simulink model "avoidance"  (R2022a)
settings: Solver=FixedStepAuto  StartTime=0.0  StopTime=15  FixedStep=0.01  RelTol=1e-3
values from neighbouring files (symbols this model uses):
  a10 = pi/4    (= 0.785398163397)    [gen_data.m]
  a20 = 3*pi/4    (= 2.35619449019)    [gen_data.m]
  x10 = x0(i,1)    [gen_data.m]
  x20 = 10+x0(i,2)    [gen_data.m]
  y10 = x0(i,3)    [gen_data.m]
  y20 = x0(i,4)    [gen_data.m]
  z0 = 0    [gen_data.m]
settings Model: Creator=diego  LastModifiedBy=diego

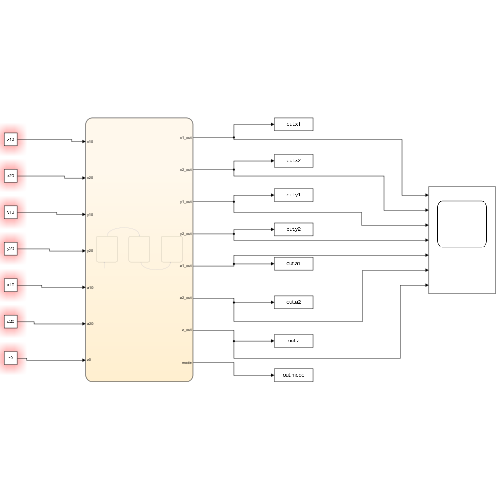
[thumbnail: Simulink's stored preview of the top-level diagram]
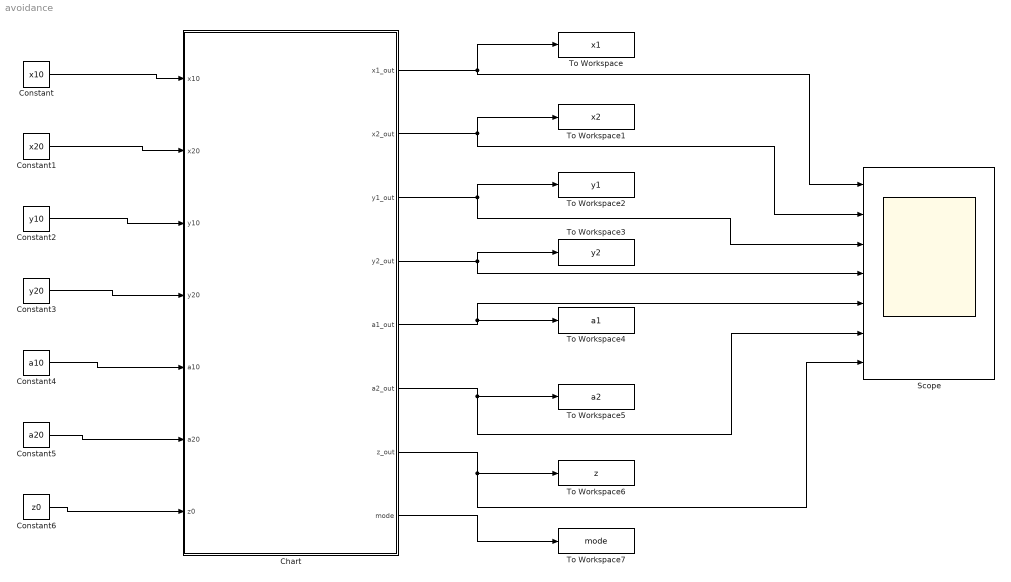
== system avoidance ==
  Chart : Stateflow chart  TreatAsAtomicUnit=on
  Constant : Constant  Value=x10
  Constant1 : Constant  Value=x20
  Constant2 : Constant  Value=y10
  Constant3 : Constant  Value=y20
  Constant4 : Constant  Value=a10
  Constant5 : Constant  Value=a20
  Constant6 : Constant  Value=z0
  Scope : Scope  NumInputPorts=7
  To Workspace : ToWorkspace  VariableName=x1  SampleTime=-1
  To Workspace1 : ToWorkspace  VariableName=x2  SampleTime=-1
  To Workspace2 : ToWorkspace  VariableName=y1  SampleTime=-1
  To Workspace3 : ToWorkspace  VariableName=y2  SampleTime=-1
  To Workspace4 : ToWorkspace  VariableName=a1  SampleTime=-1
  To Workspace5 : ToWorkspace  VariableName=a2  SampleTime=-1
  To Workspace6 : ToWorkspace  VariableName=z  SampleTime=-1
  To Workspace7 : ToWorkspace  VariableName=mode  SampleTime=-1
  wires:
  Chart/1(x1_out) -> Scope/1, To Workspace/1
  Chart/2(x2_out) -> Scope/2, To Workspace1/1
  Chart/3(y1_out) -> Scope/3, To Workspace2/1
  Chart/4(y2_out) -> Scope/4, To Workspace3/1
  Chart/5(a1_out) -> Scope/5, To Workspace4/1
  Chart/6(a2_out) -> Scope/6, To Workspace5/1
  Chart/7(z_out) -> Scope/7, To Workspace6/1
  Constant/1 -> Chart/1(x10)
  Constant6/1 -> Chart/7(z0)
  Constant5/1 -> Chart/6(a20)
  Constant4/1 -> Chart/5(a10)
  Constant3/1 -> Chart/4(y20)
  Constant2/1 -> Chart/3(y10)
  Constant1/1 -> Chart/2(x20)
  Chart/8(mode) -> To Workspace7/1

== stateflow chart avoidance/Chart ==
  settings: updateMethod=CONTINUOUS
  state Mode1
    du:
    x1_dot = cos(a1);
    x2_dot = cos(a2) ;
    y1_dot = sin(a1);
    y2_dot = sin(a2);
    z_dot = 0;
    a1_dot = 0;
    a2_dot = 0;
    x1_out = x1;
    x2_out = x2;
    y1_out = y1;
    y2_out = y2;
    a1_out = a1;
    a2_out = a2;
    z_out = z;
    mode = 1;
  state Mode2
    du:
    x1_dot = cos(a1);
    x2_dot = cos(a2) ;
    y1_dot = sin(a1);
    y2_dot = sin(a2);
    z_dot = 1;
    a1_dot = 1;
    a2_dot = 1;
    x1_out = x1;
    x2_out = x2;
    y1_out = y1;
    y2_out = y2;
    a1_out = a1;
    a2_out = a2;
    z_out = z;
    mode = 2;
  state Mode3
    du:
    x1_dot = cos(a1);
    x2_dot = cos(a2) ;
    y1_dot = sin(a1);
    y2_dot = sin(a2);
    z_dot = 0;
    a1_dot = 0;
    a2_dot = 0;
    x1_out = x1;
    x2_out = x2;
    y1_out = y1;
    y2_out = y2;
    a1_out = a1;
    a2_out = a2;
    z_out = z;
    mode = 3;
  Mode1 -> Mode2 : [(x1-x2)^2 +(y1-y2)^2 < 4]
  (default) -> Mode1 : {x1 = x10;
      | x2 = x20;
      | y1 = y10;
      | y2 = y20;
      | z = z0;
      | a1 = a10;
      | a2 = a20;}
  Mode2 -> Mode3 : [z > pi]
  data: x1_out output; x2_out output; y1_out output; y2_out output; a1_out output; a2_out output; z_out output; a1 local; a2 local; y2 local; x1 local; x2 local; y1 local; z local; x10 input; x20 input; y10 input; y20 input; a10 input; a20 input; z0 input; mode output
  data a1 settings: updateMethod=SF_CONTINUOUS_TIME_DATA
  data a2 settings: updateMethod=SF_CONTINUOUS_TIME_DATA
  data y2 settings: updateMethod=SF_CONTINUOUS_TIME_DATA
  data x1 settings: updateMethod=SF_CONTINUOUS_TIME_DATA
  data x2 settings: updateMethod=SF_CONTINUOUS_TIME_DATA
  data y1 settings: updateMethod=SF_CONTINUOUS_TIME_DATA
  data z settings: updateMethod=SF_CONTINUOUS_TIME_DATA
